simulink model "dspStartModel"  (Simulink 7.4)
settings: Solver=VariableStepDiscrete  StartTime=0  StopTime=1000  RelTol=1e-3
undefined symbols (not defined in the file or in its folder): referenceDSP
libraries: dspbuff3 x3
settings Model: Creator=Administrator  LastModifiedBy=Administrator

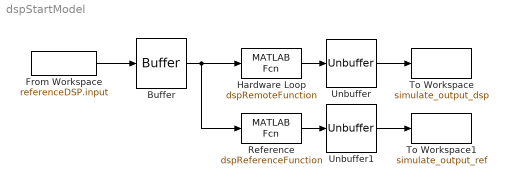
== system dspStartModel ==
  Buffer : dspbuff3/Buffer  N=referenceDSP.dspCfg.buffersize  V=0  ic=0
  From Workspace : FromWorkspace  VariableName=referenceDSP.input  SampleTime=1
  Hardware Loop : MATLABFcn  MATLABFcn=dspRemoteFunction  Output1D=off
  Reference : MATLABFcn  MATLABFcn=dspReferenceFunction  Output1D=off
  To Workspace : ToWorkspace  VariableName=simulate_output_dsp  SampleTime=-1  SaveFormat=Structure
  To Workspace1 : ToWorkspace  VariableName=simulate_output_ref  SampleTime=-1  SaveFormat=Structure
  Unbuffer : dspbuff3/Unbuffer  ic=0
  Unbuffer1 : dspbuff3/Unbuffer  ic=0
  wires:
  From Workspace/1 -> Buffer/1
  Buffer/1 -> Hardware Loop/1, Reference/1
  Hardware Loop/1 -> Unbuffer/1
  Unbuffer/1 -> To Workspace/1
  Unbuffer1/1 -> To Workspace1/1
  Reference/1 -> Unbuffer1/1
